simulink model "RWIPSimulink1axis"  (R2021b)
settings: Solver=VariableStepAuto  StartTime=0.0  StopTime=10  RelTol=1e-3
values from neighbouring files (symbols this model uses):
  g = 9.81    [pendulum.m]
  Imax = 5.6    [pendulum.m]
  Ip = 6.8E-3    (= 0.0068)    [pendulum.m]
  Iw = 6.98E-5    (= 6.98e-05)    [pendulum.m]
  Km = 7.6E-3    (= 0.0076)    [pendulum.m]
  lp = 0.077    [pendulum.m]
  lw = 0.101    [pendulum.m]
  mp = 0.1782    [pendulum.m]
  mw = 0.11528    [pendulum.m]
  x0 = [pi/30;0;0]    [pendulum.m]
  y0 = [-pi/30;0;0]    [pendulum.m]
settings Model: Creator=Utilisateur  LastModifiedBy=ryuzuu
settings SolverCC: AlgebraicLoopSolver=TrustRegion
settings DataIOCC: ReturnWorkspaceOutputs=off
settings DebuggingCC: SFMachineParentedDataDiag=warning  ArithmeticOperatorsInVariantConditions=warning
settings SFSimCC: SimUseLocalCustomCode=off  CustomCodeUndefinedFunction=UseInterfaceOnly
settings RTWCC: RTWUseLocalCustomCode=off

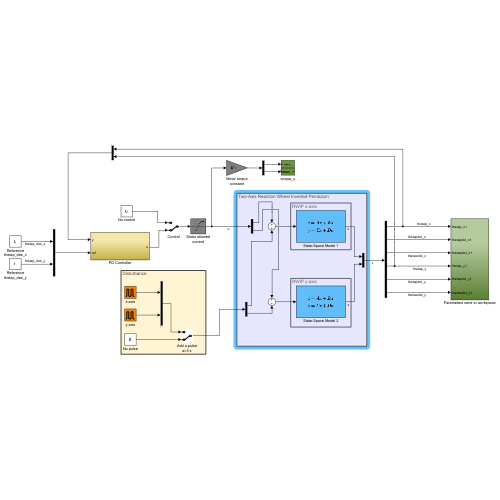
[thumbnail: Simulink's stored preview of the top-level diagram]
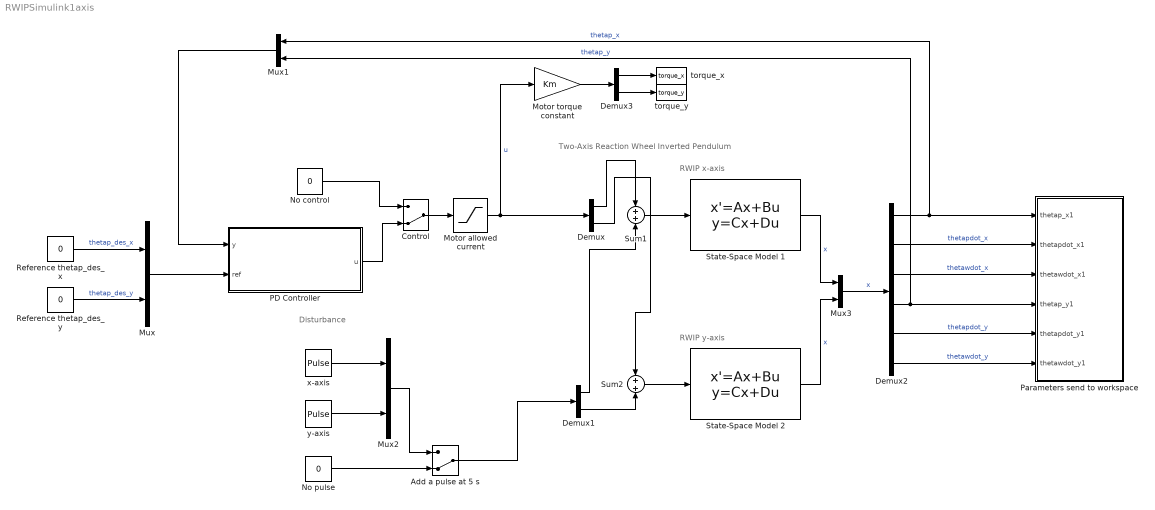
== system RWIPSimulink1axis ==
  note: RWIP y-axis
  note: RWIP x-axis
  note: Two-Axis Reaction Wheel Inverted Pendulum
  note: Disturbance
  Add a pulse at 5 s : ManualSwitch  CurrentSetting=0
  Control : ManualSwitch  CurrentSetting=0
  Demux : Demux  Outputs=2
  Demux1 : Demux  Outputs=2
  Demux2 : Demux  Outputs=6
  Demux3 : Demux  Outputs=2
  Motor allowed current : Saturate  UpperLimit=Imax  LowerLimit=-Imax
  Motor torque constant : Gain  Gain=Km
  Mux{,1..3} (4 alike) : Mux  Inputs=2
  No control : Constant  Value=0
  No pulse : Constant  Value=0
  PD Controller : Subsystem
  Parameters send to workspace : Subsystem
  Reference thetap_des_x : Constant  Value=0
  Reference thetap_des_y : Constant  Value=0
  State-Space Model 1 : StateSpace  A=[0 1 0;(mp*lp+mw*lw)*g/(mp*lp^2+mw*lw^2+Ip) 0 0;(mp*lp+mw*lw)*g/(-(mp*lp^2+mw*lw^2+Ip)) 0 0]  B=[0; -Km/(mp*lp^2+mw*lw^2+Ip); Km*(mp*lp^2+mw*lw^2+Ip+Iw)/(Iw*(mp*lp^2+mw*lw^2+Ip))]  C=eye(3)  D=[0; 0; 0]  InitialCondition=x0  ContinuousStateAttributes={'thetap', 'thetapdot', 'thetawdot'}
  State-Space Model 2 : StateSpace  A=[0 1 0;(mp*lp+mw*lw)*g/(mp*lp^2+mw*lw^2+Ip) 0 0;(mp*lp+mw*lw)*g/(-(mp*lp^2+mw*lw^2+Ip)) 0 0]  B=[0; -Km/(mp*lp^2+mw*lw^2+Ip); Km*(mp*lp^2+mw*lw^2+Ip+Iw)/(Iw*(mp*lp^2+mw*lw^2+Ip))]  C=eye(3)  D=[0; 0; 0]  InitialCondition=y0  ContinuousStateAttributes={'thetap', 'thetapdot', 'thetawdot'}
  Sum1 : Sum
  Sum2 : Sum
  torque_x : ToWorkspace  VariableName=torque_x  SaveFormat=Structure With Time  SampleTime=-1
  torque_y : ToWorkspace  VariableName=torque_y  SaveFormat=Structure With Time  SampleTime=-1
  x-axis : DiscretePulseGenerator  PulseType=Time based  Amplitude=100  Period=10  PulseWidth=0.5  PhaseDelay=5
  y-axis : DiscretePulseGenerator  PulseType=Time based  Amplitude=100  Period=10  PulseWidth=0.5  PhaseDelay=5
  wires:
  Demux2/1 -> Parameters send to workspace/1(thetap_x1), Mux1/1  "thetap_x"
  Reference thetap_des_x/1 -> Mux/1  "thetap_des_x"
  Reference thetap_des_y/1 -> Mux/2  "thetap_des_y"
  Mux2/1 -> Add a pulse at 5 s/1
  No pulse/1 -> Add a pulse at 5 s/2
  Mux3/1 -> Demux2/1  "x"
  y-axis/1 -> Mux2/2
  x-axis/1 -> Mux2/1
  Add a pulse at 5 s/1 -> Demux1/1
  Sum1/1 -> State-Space Model 1/1
  State-Space Model 1/1 -> Mux3/1  "x"
  Sum2/1 -> State-Space Model 2/1
  State-Space Model 2/1 -> Mux3/2  "x"
  Demux1/1 -> Sum1/2
  Demux1/2 -> Sum2/2
  Demux2/4 -> Parameters send to workspace/4(thetap_y1), Mux1/2  "thetap_y"
  Demux2/2 -> Parameters send to workspace/2(thetapdot_x1)  "thetapdot_x"
  Demux2/3 -> Parameters send to workspace/3(thetawdot_x1)  "thetawdot_x"
  Demux2/5 -> Parameters send to workspace/5(thetapdot_y1)  "thetapdot_y"
  Demux2/6 -> Parameters send to workspace/6(thetawdot_y1)  "thetawdot_y"
  Mux1/1 -> PD Controller/1(y)
  Mux/1 -> PD Controller/2(ref)
  No control/1 -> Control/1
  PD Controller/1(u) -> Control/2
  Control/1 -> Motor allowed current/1
  Motor allowed current/1 -> Motor torque constant/1, Demux/1  "u"
  Demux/1 -> Sum1/1
  Demux/2 -> Sum2/1
  Motor torque constant/1 -> Demux3/1
  Demux3/1 -> torque_x/1
  Demux3/2 -> torque_y/1

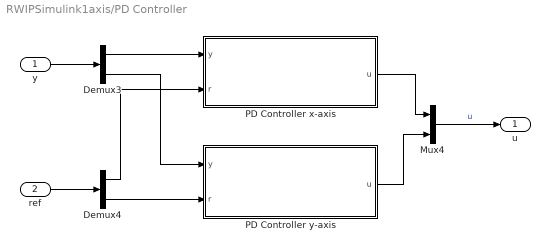
== system RWIPSimulink1axis/PD Controller ==
  y : Inport
  ref : Inport  Port=2
  Demux3 : Demux  Outputs=2
  Demux4 : Demux  Outputs=2
  Mux4 : Mux  Inputs=2
  PD Controller x-axis : Subsystem
  PD Controller y-axis : Subsystem
  u : Outport  VectorParamsAs1DForOutWhenUnconnected=off
  wires:
  ref/1 -> Demux4/1
  y/1 -> Demux3/1
  Mux4/1 -> u/1  "u"
  PD Controller x-axis/1(u) -> Mux4/1
  Demux3/1 -> PD Controller x-axis/1(y)
  Demux4/1 -> PD Controller x-axis/2(r)
  PD Controller y-axis/1(u) -> Mux4/2
  Demux4/2 -> PD Controller y-axis/2(r)
  Demux3/2 -> PD Controller y-axis/1(y)

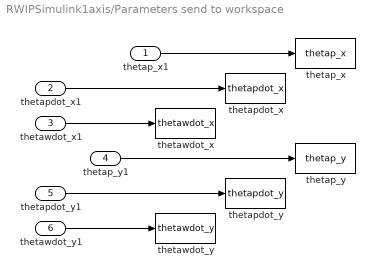
== system RWIPSimulink1axis/Parameters send to workspace ==
  thetap_x1 : Inport
  thetapdot_x1 : Inport  Port=2
  thetawdot_x1 : Inport  Port=3
  thetap_y1 : Inport  Port=4
  thetapdot_y1 : Inport  Port=5
  thetawdot_y1 : Inport  Port=6
  thetap_x : ToWorkspace  VariableName=thetap_x  SaveFormat=Structure With Time  SampleTime=-1
  thetap_y : ToWorkspace  VariableName=thetap_y  SaveFormat=Structure With Time  SampleTime=-1
  thetapdot_x : ToWorkspace  VariableName=thetapdot_x  SaveFormat=Structure With Time  SampleTime=-1
  thetapdot_y : ToWorkspace  VariableName=thetapdot_y  SaveFormat=Structure With Time  SampleTime=-1
  thetawdot_x : ToWorkspace  VariableName=thetawdot_x  SaveFormat=Structure With Time  SampleTime=-1
  thetawdot_y : ToWorkspace  VariableName=thetawdot_y  SaveFormat=Structure With Time  SampleTime=-1
  wires:
  thetapdot_y1/1 -> thetapdot_y/1
  thetapdot_x1/1 -> thetapdot_x/1
  thetawdot_y1/1 -> thetawdot_y/1
  thetawdot_x1/1 -> thetawdot_x/1
  thetap_x1/1 -> thetap_x/1
  thetap_y1/1 -> thetap_y/1

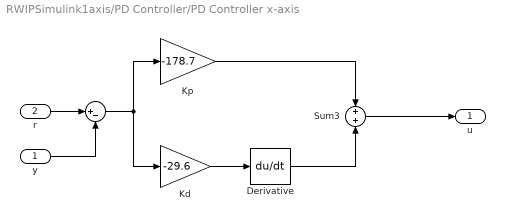
== system RWIPSimulink1axis/PD Controller/PD Controller x-axis ==
  y : Inport
  r : Inport  Port=2
  " " : Sum  Inputs=|+-
  Derivative : Derivative
  Kd : Gain  Gain=-29.6
  Kp : Gain  Gain=-178.7
  Sum3 : Sum
  u : Outport  VectorParamsAs1DForOutWhenUnconnected=off
  wires:
  Derivative/1 -> Sum3/2
  Kp/1 -> Sum3/1
  Kd/1 -> Derivative/1
  r/1 -> " "/1
  y/1 -> " "/2
  " "/1 -> Kd/1, Kp/1
  Sum3/1 -> u/1

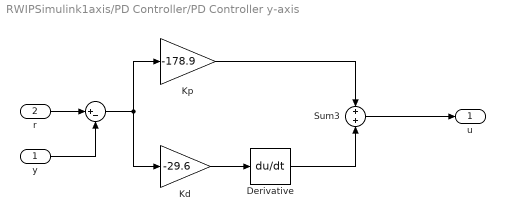
== system RWIPSimulink1axis/PD Controller/PD Controller y-axis ==
  y : Inport
  r : Inport  Port=2
  " " : Sum  Inputs=|+-
  Derivative : Derivative
  Kd : Gain  Gain=-29.6
  Kp : Gain  Gain=-178.9
  Sum3 : Sum
  u : Outport  VectorParamsAs1DForOutWhenUnconnected=off
  wires:
  Sum3/1 -> u/1
  r/1 -> " "/1
  " "/1 -> Kd/1, Kp/1
  Kd/1 -> Derivative/1
  Derivative/1 -> Sum3/2
  y/1 -> " "/2
  Kp/1 -> Sum3/1
